simulink model "arm_sim_obs"  (Simulink 7.5)
settings: Solver=ode45  StartTime=0.0  StopTime=100  RelTol=1e-3
undefined symbols (not defined in the file or in its folder): arm_ctrl_ekf, drawArm, P
libraries: simulink x1
settings Model: Creator=beard  LastModifiedBy=beard
settings OptimizationCC: InitFltsAndDblsToZero=on
settings DebuggingCC: StrictBusMsg=Warning

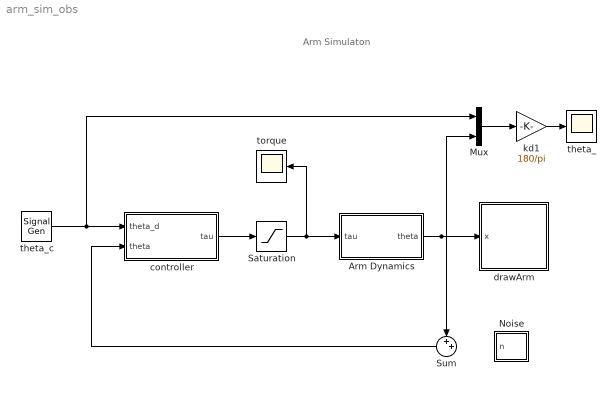
== system arm_sim_obs ==
  note: Arm Simulaton
  Arm Dynamics : Subsystem
  Mux : Mux  Inputs=2
  Noise : Subsystem
  Saturation : Saturate  UpperLimit=P.tau_max  LowerLimit=-P.tau_max
  Sum : Sum  Inputs=++|
  controller : Subsystem
  drawArm : Subsystem
      mask init:
      | % drawing parameters
      | L = 1;
      | w = 0.3;
      mask Display: image(imread('tv.jpg'))
  kd1 : Gain  Gain=180/pi
  theta_ : Scope
      settings: YMin=-75  YMax=125
  theta_c : SignalGenerator  WaveForm=square  Amplitude=25*pi/180  Frequency=.05
  torque : Scope
      settings: YMin=-0.1  YMax=1
  wires:
  Mux/1 -> kd1/1
  kd1/1 -> theta_/1
  controller/1(tau) -> Saturation/1
  theta_c/1 -> controller/1(theta_d), Mux/1
  Arm Dynamics/1(theta) -> drawArm/1(x), Mux/2, Sum/1
  Sum/1 -> controller/2(theta)
  Saturation/1 -> torque/1, Arm Dynamics/1(tau)

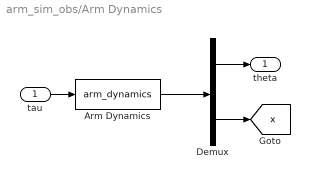
== system arm_sim_obs/Arm Dynamics ==
  tau : Inport
  Arm Dynamics : S-Function  FunctionName=arm_dynamics  Parameters=AP  EnableBusSupport=off
  Demux : Demux  Outputs=[1;2]
  theta : Outport
  tag scope: x=global
  wires:
  tau/1 -> Arm Dynamics/1
  Arm Dynamics/1 -> Demux/1
  Demux/1 -> theta/1
  Demux/2 -> [x]

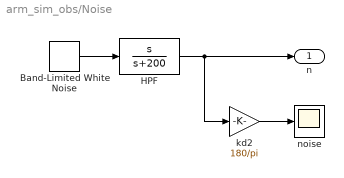
== system arm_sim_obs/Noise ==
  Band-Limited White Noise : simulink/Sources/Band-Limited White Noise  SystemSampleTime=-1  Cov=[0.000001]  Ts=P.Ts  seed=[23341]
  HPF : TransferFcn  Numerator=[1 0]  Denominator=[1 200]
  kd2 : Gain  Gain=180/pi
  noise : Scope
      settings: YMin=-7  YMax=8  SaveName=ScopeData2
  n : Outport
  wires:
  Band-Limited White Noise/1 -> HPF/1
  kd2/1 -> noise/1
  HPF/1 -> kd2/1, n/1

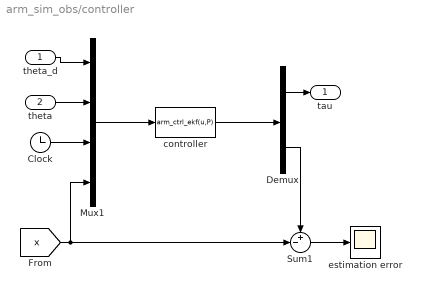
== system arm_sim_obs/controller ==
  theta_d : Inport
  theta : Inport  Port=2
  Clock : Clock
      settings: Decimation=10
  Demux : Demux  Outputs=[1;2]
  Mux1 : Mux
  Sum1 : Sum  Inputs=+-|
  controller : MATLABFcn  MATLABFcn=arm_ctrl_ekf(u,P)  OutputDimensions=1+2  SampleTime=P.Ts
  estimation error : Scope
      settings: YMin=-11  YMax=9  SaveName=ScopeData4
  tau : Outport
  wires:
  Mux1/1 -> controller/1
  theta_d/1 -> Mux1/1
  theta/1 -> Mux1/2
  Clock/1 -> Mux1/3
  controller/1 -> Demux/1
  Demux/1 -> tau/1
  Demux/2 -> Sum1/1
  Sum1/1 -> estimation error/1
  [x] -> Sum1/2, Mux1/4

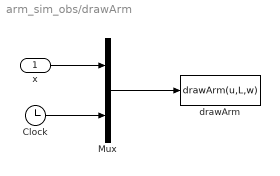
== system arm_sim_obs/drawArm ==
  x : Inport
  Clock : Clock
      settings: Decimation=10
  Mux : Mux  Inputs=2
  drawArm : MATLABFcn  MATLABFcn=drawArm(u,L,w)  OutputDimensions=0  SampleTime=0.1
  wires:
  Mux/1 -> drawArm/1
  x/1 -> Mux/1
  Clock/1 -> Mux/2
